simulink model "vehicle_animation_sim"  (Simulink 9.2)
settings: Solver=ode5  StartTime=0.0  StopTime=130  FixedStep=0.1  RelTol=1e-3
values from neighbouring files (symbols this model uses):
  vehicle_length = 2.5    [setup.m]
  X_ic = pathX(1)    [setup.m]
  Y_ic = pathY(1)    [setup.m]
  yaw_ic = atan2((pathY(2)-pathY(1)),(pathX(2)-pathX(1)))    [setup.m]
undefined symbols (not defined in the file): animation_update_interval, datetime, enable_CG_trace, enable_rearAxle_trace, plotAxisLimitMode, plotAxisLimits, save_anim_frames, vehicle_width
settings Model: Creator=comperem  LastModifiedBy=Menson
settings DataIOCC: SignalLoggingSaveFormat=Dataset
settings OptimizationCC: BlockReduction=off  BooleanDataType=off
settings DebuggingCC: SaveWithParameterizedLinksMsg=none  SignalResolutionControl=TryResolveAllWithWarning  FcnCallInpInsideContextMsg=error  AllowSymbolicDim=off  StateNameClashWarn=none
settings HardwareCC: TargetUnknown=on
settings GRTTargetCC: CombineOutputUpdateFcns=on  GRTInterface=off
settings ConfigComp: CovSFcnEnable=off

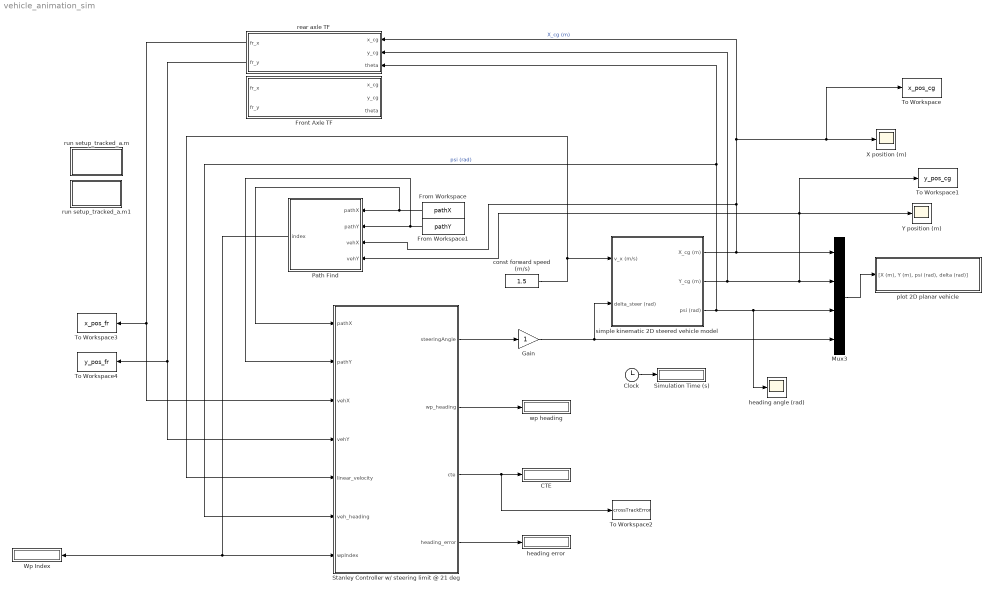
== system vehicle_animation_sim ==
  "CTE " : Display
  Clock : Clock
  From Workspace : FromWorkspace  VariableName=pathX  SampleTime=0
  From Workspace1 : FromWorkspace  VariableName=pathY  SampleTime=0
  Front Axle TF : MATLAB Function  TreatAsAtomicUnit=on
  Gain : Gain
  Mux3 : Mux
  Path Find : MATLAB Function  TreatAsAtomicUnit=on
  Simulation Time (s) : Display
  Stanley Controller w/ steering limit @ 21 deg : MATLAB Function  TreatAsAtomicUnit=on
  To Workspace : ToWorkspace  VariableName=x_pos_cg  SampleTime=-1
      settings: Save2DSignal=2-D array (concatenate along first dimension)
  To Workspace1 : ToWorkspace  VariableName=y_pos_cg  SampleTime=-1
      settings: Save2DSignal=2-D array (concatenate along first dimension)
  To Workspace2 : ToWorkspace  VariableName=crossTrackError  SampleTime=-1
      settings: Save2DSignal=2-D array (concatenate along first dimension)
  To Workspace3 : ToWorkspace  VariableName=x_pos_fr  SampleTime=-1
      settings: Save2DSignal=2-D array (concatenate along first dimension)
  To Workspace4 : ToWorkspace  VariableName=y_pos_fr  SampleTime=-1
      settings: Save2DSignal=2-D array (concatenate along first dimension)
  Wp Index : Display
  X position (m) : Scope
  Y position (m) : Scope
  const forward speed (m/s) : Constant  Value=1.5
  heading angle (rad) : Scope
  heading error : Display
  plot 2D planar vehicle : Subsystem  mask(6DoF Animation){axisMode=plotAxisLimitMode, ax=plotAxisLimits, Ts=animation_update_interval, enable_CG_trace=enable_CG_trace, enable_rearAxle_trace=enable_rearAxle_trace, save_anim_frames=save_anim_frames, anim_frame_name_str=char(datetime('now','Format','yyyy-MM-dd_HH_mm_ss')), L=vehicle_length, W=vehicle_width}
      mask prompts: axisMode "Axis Mode (0->auto, 1->fixed, BOTH use Axes Limits below)"; ax "Axes limits [xmin xmax ymin ymax] (m):"; Ts "Time interval between updates (s):"; enable_CG_trace "Enable vehicle CG trace? (0/1)"; enable_rearAxle_trace "Enable rear axle trace? (0/1)"; save_anim_frames "Save animaton frames? (0/1)"; anim_frame_name_str "Animation sequence name (if save frames==1)"; L "Vehicle length (m)"; W "Vehicle width (m)"
      mask help:
      | Create a 2D animated view of a steering vehicle model with tires.
      |
      | Marc Compere
      | CompereM@saic.com
      | created : 22 August 2002
      | modified: 28 Dec 2015
      mask init:
      | Config.axisMode=axisMode;
      | Config.ax=ax;
      | Config.Ts=Ts;
      | Config.enable_CG_trace=enable_CG_trace;
      | Config.enable_rearAxle_trace=enable_rearAxle_trace;
      | Config.save_anim_frames=save_anim_frames;
      | Config.anim_frame_name_str=anim_frame_name_str;
      | Config.L=L;
      | Config.W=W;
      mask Help:
      | <p>This block generates a 3 dimensional display of a simulation trajectory, with the craft orientation displayed during flight</p>
      | 
      | <p>There are two inputs to this block, Position and Euler.  These inputs contain more than one signal as described below.</p>
      | 
      | <p><H4>Block Vector Input - Position</H4>
      | <ul>
      | <li>X Position</li>
      | <li>Y Position</li>
      | <li>Z Position</li>
      | </ul>
      | </p>
      | 
      | <p><H4>Block Vector Input - Euler</H4>
      |     <ul>
      |     <li>Roll Attitude</li>
      |     <li>Pitch Attitude</li>
      |     <li>Yaw Attitude</li>
      |    </ul>
      |    </p>
  rear axle TF : MATLAB Function  TreatAsAtomicUnit=on
  run setup_tracked_a.m : Subsystem
      settings: OpenFcn=setup
      mask Display: fprintf('run setup.m')
  run setup_tracked_a.m1 : Subsystem
      settings: OpenFcn=edit setup
      mask Display: fprintf('edit setup.m')
  simple kinematic 2D steered vehicle model : Subsystem
  wp heading : Display
  wires:
  simple kinematic 2D steered vehicle model/1(X_cg (m)) -> rear axle TF/1(x_cg), To Workspace/1, X position (m)/1, Path Find/3(vehX), Mux3/1  "X_cg (m)"
  simple kinematic 2D steered vehicle model/2(Y_cg (m)) -> rear axle TF/2(y_cg), Path Find/4(vehY), Y position (m)/1, To Workspace1/1, Mux3/2
  simple kinematic 2D steered vehicle model/3(psi (rad)) -> Stanley Controller w/ steering limit @ 21 deg/6(veh_heading), rear axle TF/3(theta), heading angle (rad)/1, Mux3/3  "psi (rad)"
  Clock/1 -> Simulation Time (s)/1
  Mux3/1 -> plot 2D planar vehicle/1("[X (m), Y (m), psi (rad), delta (rad)]")
  const forward speed (m/s)/1 -> Stanley Controller w/ steering limit @ 21 deg/5(linear_velocity), simple kinematic 2D steered vehicle model/1(v_x (m/s))
  Gain/1 -> simple kinematic 2D steered vehicle model/2(delta_steer (rad)), Mux3/4
  Stanley Controller w/ steering limit @ 21 deg/1(steeringAngle) -> Gain/1
  Path Find/1(index) -> Stanley Controller w/ steering limit @ 21 deg/7(wpIndex), Wp Index/1
  Stanley Controller w/ steering limit @ 21 deg/2(wp_heading) -> wp heading/1
  Stanley Controller w/ steering limit @ 21 deg/3(cte) -> To Workspace2/1, "CTE "/1
  Stanley Controller w/ steering limit @ 21 deg/4(heading_error) -> heading error/1
  From Workspace/1 -> Stanley Controller w/ steering limit @ 21 deg/1(pathX), Path Find/1(pathX)
  From Workspace1/1 -> Stanley Controller w/ steering limit @ 21 deg/2(pathY), Path Find/2(pathY)
  rear axle TF/1(fr_x) -> To Workspace3/1, Stanley Controller w/ steering limit @ 21 deg/3(vehX)
  rear axle TF/2(fr_y) -> To Workspace4/1, Stanley Controller w/ steering limit @ 21 deg/4(vehY)

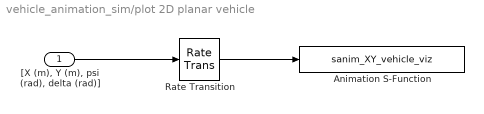
== system vehicle_animation_sim/plot 2D planar vehicle ==
  "[X (m), Y (m), psi (rad), delta (rad)]" : Inport
  Animation S-Function : S-Function  FunctionName=sanim_XY_vehicle_viz  Parameters=Config  SFunctionDeploymentMode=off  EnableBusSupport=off
  Rate Transition : RateTransition  Integrity=off
  wires:
  "[X (m), Y (m), psi (rad), delta (rad)]"/1 -> Rate Transition/1
  Rate Transition/1 -> Animation S-Function/1

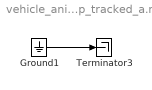
== system vehicle_animation_sim/run setup_tracked_a.m ==
  Ground1 : Ground
  Terminator3 : Terminator
  wires:
  Ground1/1 -> Terminator3/1

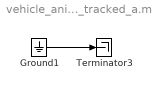
== system vehicle_animation_sim/run setup_tracked_a.m1 ==
  Ground1 : Ground
  Terminator3 : Terminator
  wires:
  Ground1/1 -> Terminator3/1

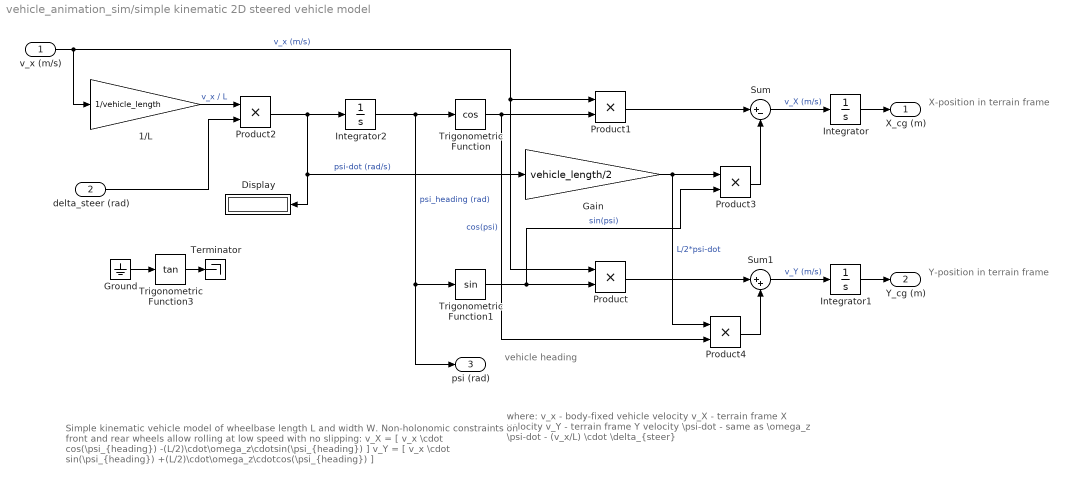
== system vehicle_animation_sim/simple kinematic 2D steered vehicle model ==
  note: where:
      |    v_x - body-fixed vehicle velocity
      |    v_X - terrain frame X velocity
      |    v_Y - terrain frame Y velocity
      |    \psi-dot - same as \omega_z
      |    \psi-dot - (v_x/L) \cdot \delta_{steer}
  note: X-position in
      | terrain frame
  note: Simple kinematic vehicle model of wheelbase
      | length L and width W.
      | Non-holonomic constraints on front and rear wheels
      | allow rolling at low speed with no slipping:
      |
      |    v_X = [ v_x \cdot cos(\psi_{heading}) -(L/2)\cdot\omega_z\cdotsin(\psi_{heading}) ]
      |    v_Y = [ v_x \cdot sin(\psi_{heading}) +(L/2)\cdot\omega_z\cdotcos(\psi_{heading}) ]
  note: vehicle
      | heading
  note: Y-position in
      | terrain frame
  v_x (m/s) : Inport
  delta_steer (rad) : Inport  Port=2
  1/L : Gain  Gain=1/vehicle_length
  Display : Display
  Gain : Gain  Gain=vehicle_length/2
  Ground : Ground
  Integrator : Integrator  InitialCondition=X_ic
  Integrator1 : Integrator  InitialCondition=Y_ic
  Integrator2 : Integrator  InitialCondition=yaw_ic
  Product{,1..4} (5 alike) : Product  RndMeth=Zero
  Sum : Sum  Inputs=|+-
  Sum1 : Sum  Inputs=|++
  Terminator : Terminator
  Trigonometric Function : Trigonometry  Operator=cos
  Trigonometric Function1 : Trigonometry
  Trigonometric Function3 : Trigonometry  Operator=tan
  X_cg (m) : Outport  OutDataTypeStr=double  PortDimensions=1
  Y_cg (m) : Outport  Port=2  OutDataTypeStr=double  PortDimensions=1
  psi (rad) : Outport  Port=3
  wires:
  Product/1 -> Sum1/1
  Product1/1 -> Sum/1
  Trigonometric Function/1 -> Product4/2, Product1/2  "cos(psi)"
  Trigonometric Function1/1 -> Product/2, Product3/2  "sin(psi)"
  Integrator2/1 -> Trigonometric Function/1, Trigonometric Function1/1, psi (rad)/1  "psi_heading (rad)"
  Integrator/1 -> X_cg (m)/1
  Integrator1/1 -> Y_cg (m)/1
  v_x (m/s)/1 -> Product/1, Product1/1, 1/L/1  "v_x (m/s)"
  Product2/1 -> Gain/1, Display/1, Integrator2/1  "psi-dot (rad/s)"
  1/L/1 -> Product2/1  "v_x / L"
  Sum/1 -> Integrator/1  "v_X (m/s)"
  Sum1/1 -> Integrator1/1  "v_Y (m/s)"
  Gain/1 -> Product4/1, Product3/1  "L/2*psi-dot"
  Product3/1 -> Sum/2
  Product4/1 -> Sum1/2
  delta_steer (rad)/1 -> Product2/2
  Ground/1 -> Trigonometric Function3/1
  Trigonometric Function3/1 -> Terminator/1

== matlab function Path Find ==
  data: pathX input double; pathY input double; vehX input double; vehY input double; index output double size=1
function index = path(pathX,pathY,vehX,vehY)
index = pathSearch(pathX,pathY,vehX,vehY);
end

== matlab function Stanley Controller w// steering limit @ 21 deg ==
  data: pathX input double; steeringAngle output double; pathY input double; vehX input double size=1; vehY input double size=1; linear_velocity input double; veh_heading input double; wpIndex input double; wp_heading output double; cte output double; heading_error output double
function [steeringAngle, wp_heading, cte, heading_error] = stanley(pathX,pathY,vehX,vehY,linear_velocity,veh_heading, wpIndex)
    [steeringAngle,wp_heading, cte, heading_error] = stanleyController(pathX,pathY,vehX,vehY,linear_velocity,veh_heading, wpIndex);
end

== matlab function Front Axle TF ==
  data: x_cg input double; fr_x output double; fr_y output double; y_cg input double; theta input double
function [fr_x, fr_y] = cg_to_front_axle(x_cg, y_cg, theta)

fr_x = x_cg + (2.5*cos(theta));
fr_y = y_cg + (2.5*sin(theta));
end

== matlab function rear axle TF ==
  data: x_cg input double; fr_x output double; fr_y output double; y_cg input double; theta input double
function [fr_x, fr_y] = cg_to_rear_axle(x_cg, y_cg, theta)

fr_x = x_cg - (2.5*cos(theta));
fr_y = y_cg - (2.5*sin(theta));
end
